simulink model "chap2_sim"  (R2025b)
settings: Solver=ode4  StartTime=0.0  StopTime=1  FixedStep=0.02  RelTol=1e-3
settings Model: Creator=ASUS  LastModifiedBy=ASUS

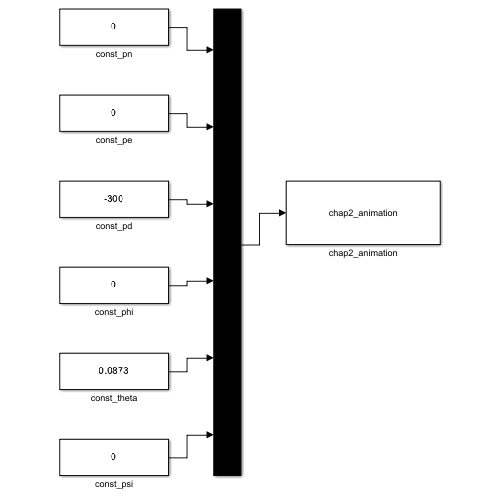
[thumbnail: Simulink's stored preview of the top-level diagram]
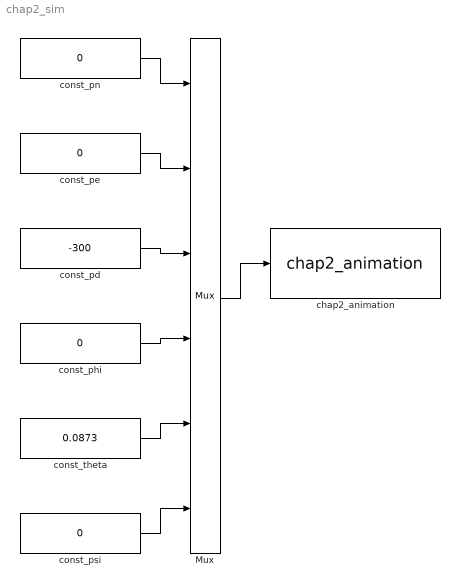
== system chap2_sim ==
  Mux : Mux  Inputs=6
  chap2_animation : M-S-Function  FunctionName=chap2_animation  Parameters=1
  const_pd : Constant  Value=-300  OutDataTypeStr=double
  const_pe : Constant  Value=0  OutDataTypeStr=double
  const_phi : Constant  Value=0  OutDataTypeStr=double
  const_pn : Constant  Value=0  OutDataTypeStr=double
  const_psi : Constant  Value=0  OutDataTypeStr=double
  const_theta : Constant  Value=0.0873  OutDataTypeStr=double
  wires:
  const_pn/1 -> Mux/1
  const_pe/1 -> Mux/2
  const_pd/1 -> Mux/3
  const_phi/1 -> Mux/4
  const_theta/1 -> Mux/5
  const_psi/1 -> Mux/6
  Mux/1 -> chap2_animation/1
